simulink model "RealHardwareControlNull"  (R2015a)
settings: configuration reference "SIMULATION_CONFIGURATION" (kept outside this file)
settings Model: Creator=moritz  LastModifiedBy=moritz
settings ConfigSetRef: SourceLocation=Base Workspace

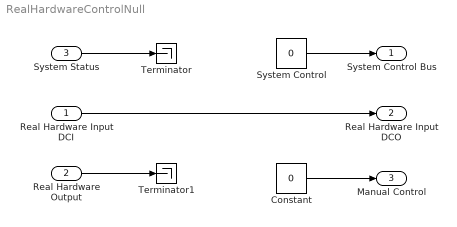
== system RealHardwareControlNull ==
  Real Hardware Input DCI : Inport  OutDataTypeStr=Bus: HARDWARE_IO_INPUT_BUS  BusOutputAsStruct=on
  Real Hardware Output : Inport  Port=2  OutDataTypeStr=Bus: HARDWARE_IO_OUTPUT_BUS
  System Status : Inport  Port=3
  Constant : Constant  Value=0  OutDataTypeStr=boolean
  System Control : Constant  Value=0  OutDataTypeStr=Bus: SYSTEM_CONTROL_BUS
  Terminator : Terminator
  Terminator1 : Terminator
  System Control Bus : Outport  OutDataTypeStr=Bus: SYSTEM_CONTROL_BUS  BusOutputAsStruct=on
  Real Hardware Input DCO : Outport  Port=2  OutDataTypeStr=Bus: HARDWARE_IO_INPUT_BUS  BusOutputAsStruct=on
  Manual Control : Outport  Port=3
  wires:
  Constant/1 -> Manual Control/1
  System Control/1 -> System Control Bus/1
  System Status/1 -> Terminator/1
  Real Hardware Input DCI/1 -> Real Hardware Input DCO/1
  Real Hardware Output/1 -> Terminator1/1
